simulink model "IMUparam"  (R2018b)
settings: Solver=VariableStepAuto  StartTime=0.0  StopTime=10.0  RelTol=1e-3
undefined symbols (not defined in the file or in its folder): ba, bg
libraries: simulink x1, aerolibnav x1
settings Model: Creator=Ares  LastModifiedBy=Ares

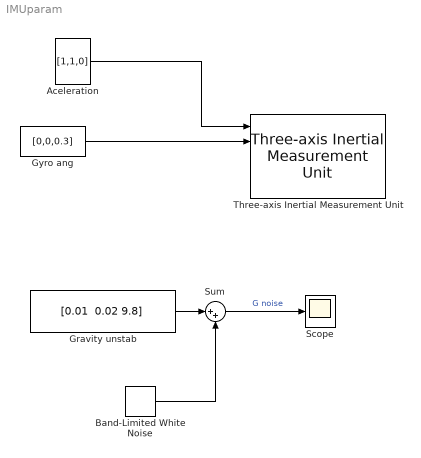
== system IMUparam ==
  Aceleration : Constant  Value=[1,1,0]
  Band-Limited White Noise : simulink/Sources/Band-Limited White Noise  Cov=[0.001]  Ts=0.01  seed=[23341]
  Gravity unstab : Constant  Value="[0.01  0.02 9.8]"
  Gyro ang : Constant  Value=[0,0,0.3]
  Scope : Scope
  Sum : Sum  Inputs=|++
  Three-axis Inertial Measurement Unit : aerolibnav/Three-axis Inertial Measurement Unit  units=Metric (MKS)  imu=[0 0 0]  i_Ts=0  dtype_a=on  w_a=190  z_a=0.707  a_sf_cc=[1 0 0; 0 1 0; 0 0 1]  a_bias=[ba ba ba]  a_sat="[-inf  -inf  -inf  inf inf inf]"  dtype_g=on  w_g=190  z_g=0.707  g_sf_cc=[1 0 0; 0 1 0; 0 0 1]  g_bias=[bg bg bg]  g_sens=[0 0 0]  g_sat="[-inf  -inf  -inf  inf inf inf]"  i_rand=on  i_seeds=[23093 23094 23095 23096 23097 23098]  i_pow=[0.001 0.001 0.001 0.0001 0.0001 0.0001]
  wires:
  Aceleration/1 -> Three-axis Inertial Measurement Unit/1
  Gyro ang/1 -> Three-axis Inertial Measurement Unit/2
  Band-Limited White Noise/1 -> Sum/2
  Sum/1 -> Scope/1  "G noise"
  Gravity unstab/1 -> Sum/1
